simulink model "Scratch_SIMULATION_02"  (R2016a)
settings: Solver=VariableStepAuto  StartTime=0.0  StopTime=3  RelTol=1e-3
undefined symbols (not defined in the file or in its folder): sigbuilder_block
settings Model: Creator=Dell  LastModifiedBy=Dell

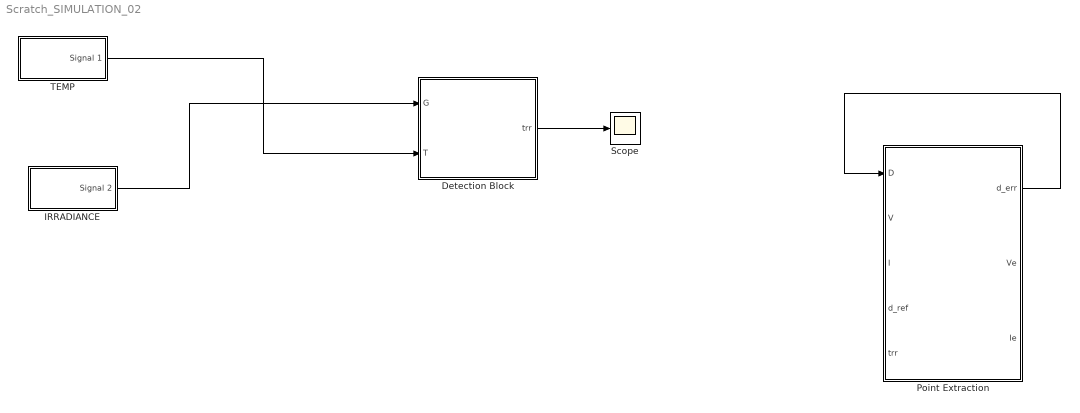
== system Scratch_SIMULATION_02 ==
  Detection Block : MATLAB Function  TreatAsAtomicUnit=on
  IRRADIANCE : Subsystem  Tag=STV Subsys  LoadFcn=sigbuilder_block('load');  StartFcn=sigbuilder_block('start');  StopFcn=sigbuilder_block('stop');  ClipboardFcn=sigbuilder_block('clipboard');  mask(Sigbuilder block){}
      mask help: Simulink:masks:SigbuilderBlock_MD
      mask init:
      | if ~strcmp(get_param(bdroot(gcbh),'SimulationStatus'),'stopped') tuvar = sigbuilder_block('maskInit'); end
      settings: CopyFcn=sigbuilder_block('copy');  DeleteFcn=sigbuilder_block('delete');  ModelCloseFcn=sigbuilder_block('modelClose');  PreSaveFcn=sigbuilder_block('preSave');  PauseFcn=sigbuilder_block('pause');  ContinueFcn=sigbuilder_block('continue');  NameChangeFcn=sigbuilder_block('namechange');  OpenFcn=sigbuilder_block('open',[0.6 0.6 574.8 585.6 ]);  CloseFcn=sigbuilder_block('close');
      mask Display: plot(0, 0, 100, 100,[2, 2, 32, 32, 2], [68, 8, 8, 68, 68],[32, 2], [38, 38], [32, 19, 2],[53, 60, 44], [32, 17, 17, 2],[16, 16, 31, 31]);txt = getActiveGroup(gcbh);text(2, 100, txt,'verticalAlignment', 'top');
  Point Extraction : MATLAB Function  TreatAsAtomicUnit=on
  Scope : Scope
  TEMP : Subsystem  Tag=STV Subsys  LoadFcn=sigbuilder_block('load');  StartFcn=sigbuilder_block('start');  StopFcn=sigbuilder_block('stop');  ClipboardFcn=sigbuilder_block('clipboard');  mask(Sigbuilder block){}
      mask help: Simulink:masks:SigbuilderBlock_MD
      mask init:
      | if ~strcmp(get_param(bdroot(gcbh),'SimulationStatus'),'stopped') tuvar = sigbuilder_block('maskInit'); end
      settings: CopyFcn=sigbuilder_block('copy');  DeleteFcn=sigbuilder_block('delete');  ModelCloseFcn=sigbuilder_block('modelClose');  PreSaveFcn=sigbuilder_block('preSave');  PauseFcn=sigbuilder_block('pause');  ContinueFcn=sigbuilder_block('continue');  NameChangeFcn=sigbuilder_block('namechange');  OpenFcn=sigbuilder_block('open',[6 28.2 1012.8 484.8 ]);  CloseFcn=sigbuilder_block('close');
      mask Display: plot(0, 0, 100, 100,[2, 2, 32, 32, 2], [68, 8, 8, 68, 68],[32, 2], [38, 38], [32, 19, 2],[53, 60, 44], [32, 17, 17, 2],[16, 16, 31, 31]);txt = getActiveGroup(gcbh);text(2, 100, txt,'verticalAlignment', 'top');
  wires:
  TEMP/1(Signal 1) -> Detection Block/2(T)
  IRRADIANCE/1(Signal 2) -> Detection Block/1(G)
  Detection Block/1(trr) -> Scope/1
  Point Extraction/1(d_err) -> Point Extraction/1(D)

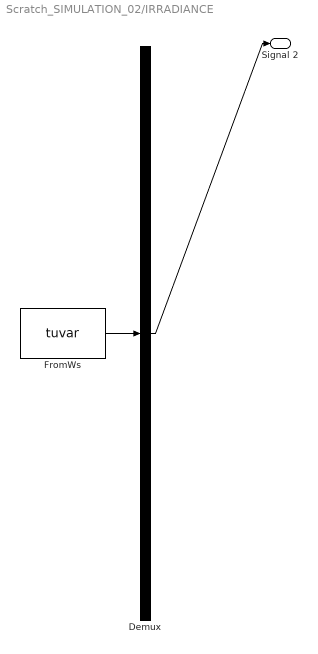
== system Scratch_SIMULATION_02/IRRADIANCE ==
  Demux : Demux  Tag=STV Demux  Outputs=1
  FromWs : FromWorkspace  Tag=STV FromWs  VariableName=tuvar  SampleTime=0
      SigBuilderData=|
      | common.afterFinalStr = 'Extrapolate'
      | common.sampleTime = 0
      | dataSet.timeRange = [0 10]
      | dataSet.name = 'Group 1'
      | sbobj.Groups.Name = 'Group 1'
      | sbobj.Groups.Signals.Name = 'Signal 2'
      | sbobj.Groups.Signals.XData = [0 1 1 1.5 1.5 2 2 2.5 2.5 10]
      | sbobj.Groups.Signals.YData = [1 1 0.8 0.8 0.7 0.7 0.5 0.5 1 1]
  Signal 2 : Outport  Tag=STV Outport
  wires:
  FromWs/1 -> Demux/1
  Demux/1 -> Signal 2/1

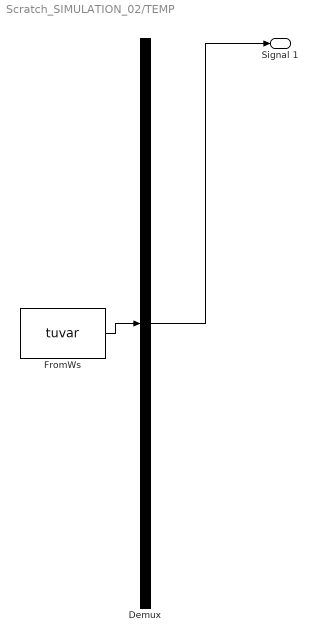
== system Scratch_SIMULATION_02/TEMP ==
  Demux : Demux  Tag=STV Demux  Outputs=1
  FromWs : FromWorkspace  Tag=STV FromWs  VariableName=tuvar  SampleTime=0
      SigBuilderData=|
      | common.afterFinalStr = 'Extrapolate'
      | common.sampleTime = 0
      | dataSet.timeRange = [0 10]
      | dataSet.name = 'Group 1'
      | sbobj.Groups.Name = 'Group 1'
      | sbobj.Groups.Signals.Name = 'Signal 1'
      | sbobj.Groups.Signals.XData = [0 10]
      | sbobj.Groups.Signals.YData = [25 25]
  Signal 1 : Outport  Tag=STV Outport
  wires:
  Demux/1 -> Signal 1/1
  FromWs/1 -> Demux/1

== matlab function Scratch_SIMULATION_02/Point Extraction ==
  data: D input; d_err output; V input; I input; d_ref input; Ve output; Ie output; trr input

function [d_err,Ve,Ie]= Curve_Fitting(D ,V , I, d_ref, trr)
             
     

        persistent d_1 d_2 Vo Io io d_new
        dataType = 'double';
      
        if d_ref ~= d_new
                 vars = whos;
                vars = vars([vars.persistent]);
                varName = {vars.name};
                clear(varName{:});
                d_err=d_ref;
                Ve=[];
                Ie=[];
                return;
                
        end
    
        if isempty(Vo)
            Vo=0;
            Io=0;
            io=1;
            d_1=0;
            d_2=0;
            d_new=d_ref;
        end
        
        
        Vo
        Io
        d_ref 
        d_1
        d_2
      
                 if length(Vo)==3
                        Ve=Vo;
                        Ie=Io;
                        d_err=d_ref;
                        disp('Vector Array Limit Is Exceeded')

                        return;    
                 end

                 if length(Vo)<=2       
                        if D==d_1

                            disp('Adding Second Point in Array Vo and Io')
                            Vo(io)=V;
                            Io(io)=I;
                            d_2=d_ref - 0.2*d_ref;
                            d_err=d_2;     
                            io=io+1;

                        end

                        if D==d_ref
                            disp('Adding First Point in Array Vo and Io')
                            Vo(io)=V;
                            Io(io)=I;
                            d_1=d_ref + 0.2*d_ref;
                            d_err=d_1;
                            io=io+1;
                        end

                        if D==d_2
                            disp('Adding third Point in Array Vo and Io')
                            Vo(io)=V;
                            Io(io)=I;
                            d_err=d_2;
                            io=io+1;

                        end 
                 end
        
        Ve=Vo;
        Ie=Io;
end

== matlab function Scratch_SIMULATION_02/Detection Block ==
  data: G input; trr output; T input
function trr= Detection(G,T)

     persistent G_ref
     
     dataType = 'double';
     
      if isempty(G_ref)
          G_ref=0;
      end
      
      if G==G_ref
         
          trr=0;
          G_ref=G;
          
      else
          
          trr=1;
          G_ref=G;
          
      
      end 



end
